simulink model "SIMULACIO_BATERIA"  (R2020b)
settings: Solver=VariableStepAuto  StartTime=0.1  StopTime=500  FixedStep=1e-4  RelTol=1e-3
values from neighbouring files (symbols this model uses):
  Guany = 0.97    [valors_model_v2.m]
  k = 1/1000000    (= 1e-06)    [valors_model_v2.m]
  P = g*d*h*n    (= 104182.2)    [valors_model_v2.m]
  R = -0.05    [valors_model_v2.m]
  tau = 0.010    (= 0.01)    [valors_model_v2.m]
libraries: simulink x4
settings Model: Creator=34691  LastModifiedBy=34691

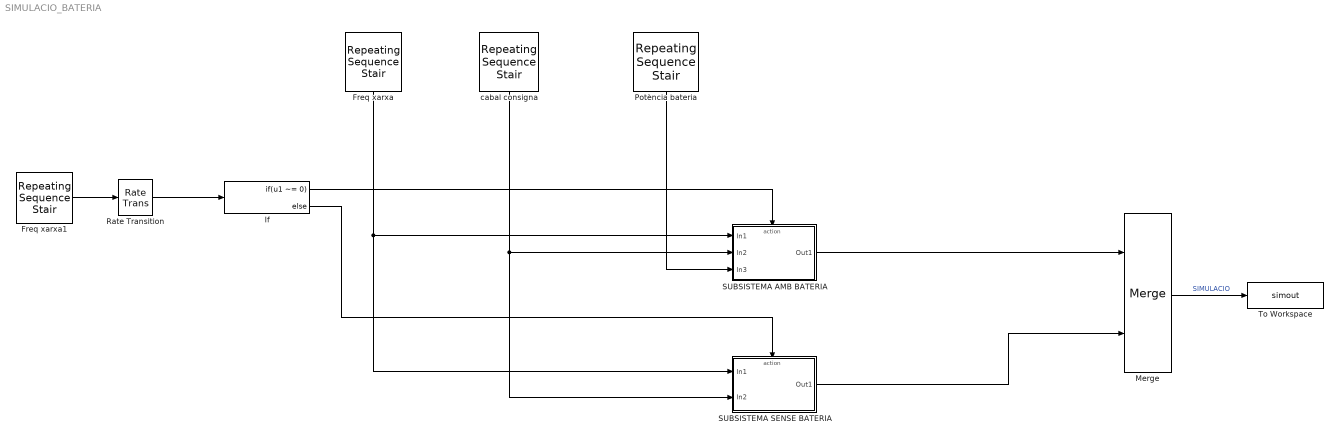
== system SIMULACIO_BATERIA ==
  Freq xarxa : simulink/Sources/Repeating Sequence Stair  OutValues=freq  tsamp=0.1  OutMin=[]  OutMax=[]  OutDataTypeStr=double  OutputDataTypeScalingMode=double  OutDataType=fixdt(0,8)  ConRadixGroup=Best Precision: Vector-wise  OutScaling=2^-12
  Freq xarxa1 : simulink/Sources/Repeating Sequence Stair  OutValues=freq  tsamp=0.1  OutMin=[]  OutMax=[]  OutDataTypeStr=double  OutputDataTypeScalingMode=double  OutDataType=fixdt(0,8)  ConRadixGroup=Best Precision: Vector-wise  OutScaling=2^-12
  If : If  IfExpression=u1 ~= 0
  Merge : Merge
  Potència bateria : simulink/Sources/Repeating Sequence Stair  OutValues=bpow  tsamp=0.1  OutMin=[]  OutMax=[]  OutDataTypeStr=double  OutputDataTypeScalingMode=double  OutDataType=fixdt(0,8)  ConRadixGroup=Best Precision: Vector-wise  OutScaling=2^-12
  Rate Transition : RateTransition
  SUBSISTEMA AMB BATERIA : Subsystem  TreatAsAtomicUnit=on
  SUBSISTEMA SENSE BATERIA : Subsystem  TreatAsAtomicUnit=on
  To Workspace : ToWorkspace  VariableName=simout  SaveFormat=Timeseries  SampleTime=-1
  cabal consigna : simulink/Sources/Repeating Sequence Stair  OutValues=cabal  tsamp=0.1  OutMin=[]  OutMax=[]  OutDataTypeStr=double  OutputDataTypeScalingMode=double  OutDataType=fixdt(0,8)  ConRadixGroup=Best Precision: Vector-wise  OutScaling=2^-12
  wires:
  SUBSISTEMA AMB BATERIA/1(Out1) -> Merge/1
  SUBSISTEMA SENSE BATERIA/1(Out1) -> Merge/2
  Freq xarxa1/1 -> Rate Transition/1
  Rate Transition/1 -> If/1
  Merge/1 -> To Workspace/1  "SIMULACIO"
  If/1 -> SUBSISTEMA AMB BATERIA/Action
  Freq xarxa/1 -> SUBSISTEMA SENSE BATERIA/1(In1), SUBSISTEMA AMB BATERIA/1(In1)
  cabal consigna/1 -> SUBSISTEMA SENSE BATERIA/2(In2), SUBSISTEMA AMB BATERIA/2(In2)
  Potència bateria/1 -> SUBSISTEMA AMB BATERIA/3(In3)
  If/2 -> SUBSISTEMA SENSE BATERIA/Action

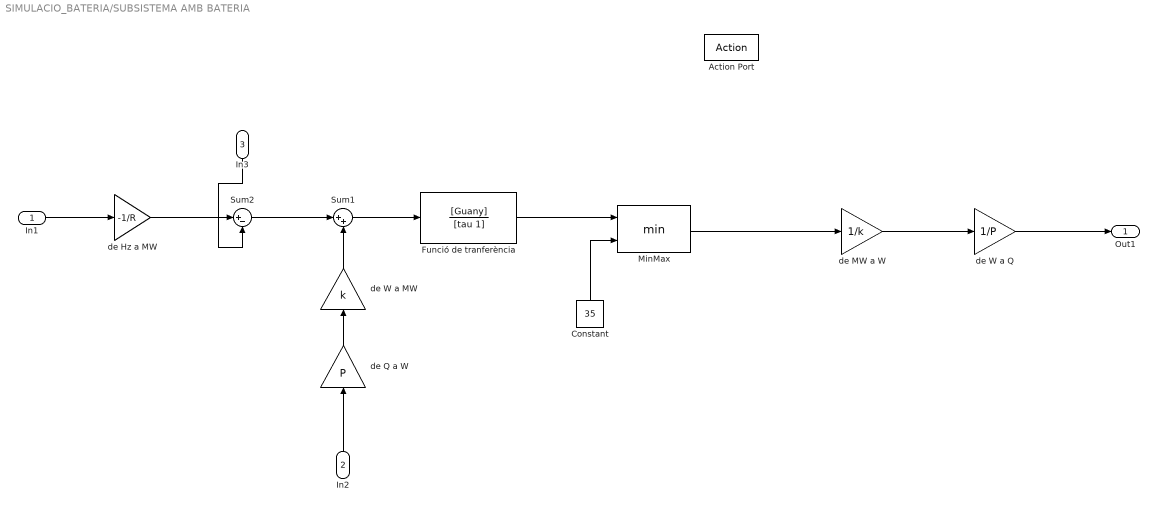
== system SIMULACIO_BATERIA/SUBSISTEMA AMB BATERIA ==
  In1 : Inport
  In2 : Inport  Port=2
  In3 : Inport  Port=3
  Action Port : ActionPort  ActionPortLabel=if(u1 ~= 0)
  Constant : Constant  Value=35
  Funció de tranferència : TransferFcn  Numerator=[Guany]  Denominator=[tau 1]
  MinMax : MinMax  Inputs=2
  Sum1 : Sum  Inputs=|++
  Sum2 : Sum  Inputs=|+-
  de Hz a MW : Gain  Gain=-1/R
  de MW a W : Gain  Gain=1/k
  de Q a W : Gain  Gain=P
  de W a MW : Gain  Gain=k
  de W a Q : Gain  Gain=1/P
  Out1 : Outport
  wires:
  Sum1/1 -> Funció de tranferència/1
  Constant/1 -> MinMax/2
  Funció de tranferència/1 -> MinMax/1
  In1/1 -> de Hz a MW/1
  de Q a W/1 -> de W a MW/1
  de W a MW/1 -> Sum1/2
  In2/1 -> de Q a W/1
  de W a Q/1 -> Out1/1
  de MW a W/1 -> de W a Q/1
  In3/1 -> Sum2/2
  de Hz a MW/1 -> Sum2/1
  Sum2/1 -> Sum1/1
  MinMax/1 -> de MW a W/1

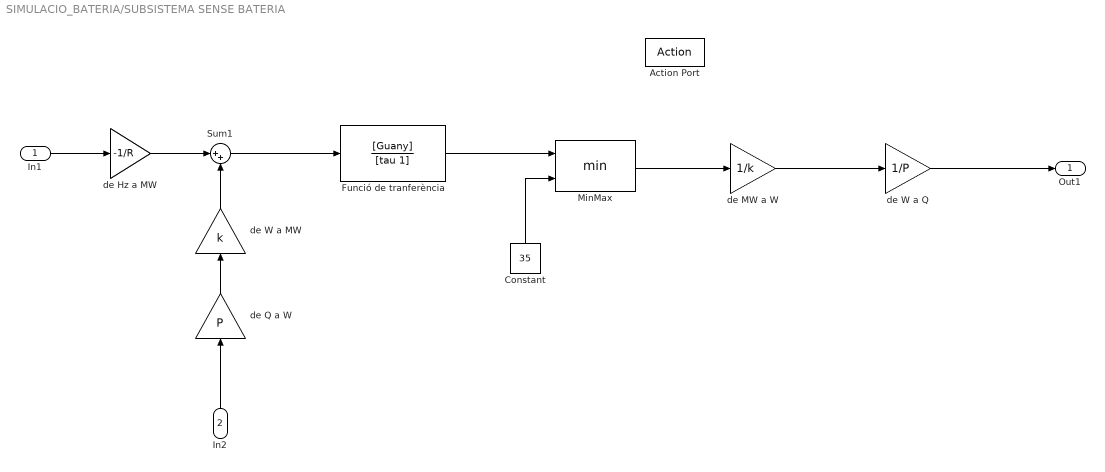
== system SIMULACIO_BATERIA/SUBSISTEMA SENSE BATERIA ==
  In1 : Inport
  In2 : Inport  Port=2
  Action Port : ActionPort  ActionPortLabel=else
  Constant : Constant  Value=35
  Funció de tranferència : TransferFcn  Numerator=[Guany]  Denominator=[tau 1]
  MinMax : MinMax  Inputs=2
  Sum1 : Sum  Inputs=|++
  de Hz a MW : Gain  Gain=-1/R
  de MW a W : Gain  Gain=1/k
  de Q a W : Gain  Gain=P
  de W a MW : Gain  Gain=k
  de W a Q : Gain  Gain=1/P
  Out1 : Outport
  wires:
  MinMax/1 -> de MW a W/1
  In2/1 -> de Q a W/1
  Sum1/1 -> Funció de tranferència/1
  In1/1 -> de Hz a MW/1
  de W a MW/1 -> Sum1/2
  de Q a W/1 -> de W a MW/1
  de MW a W/1 -> de W a Q/1
  de Hz a MW/1 -> Sum1/1
  Funció de tranferència/1 -> MinMax/1
  Constant/1 -> MinMax/2
  de W a Q/1 -> Out1/1
